simulink model "dcmotor_sim"  (R2020b)
settings: Solver=FixedStepAuto  StartTime=0.0  StopTime=40  FixedStep=Ts  MaxStep=Ts  RelTol=1e-12  AbsTol=1e-6
values from neighbouring files (symbols this model uses):
  Ad = eye(2) + A*Ts    [dcmotor.m]    (also in makedcmotorparams.m)
  Bd = B*Ts    [dcmotor.m]    (also in makedcmotorparams.m)
  C = [1, 1]    [dcmotor.m]    (also in makedcmotorparams.m; tanks.m = [0 1])
  Cd = C    [dcmotor.m]    (also in makedcmotorparams.m)
  delta = 1e-2    (= 0.01)    [dcmotor.m]    (also in makedcmotorparams.m)
  K = place(Ad, Bd, cpoles)    [dcmotor.m]    (also in makedcmotorparams.m)
  L = place(Ad', Cd', [0.6, 0.5]).'    [dcmotor.m]    (also in makedcmotorparams.m = place(Ad', Cd', [0.6, 0]).'; tanks.m = place(A', C', [-100 -2])')
  N = 1/(0.784815)    (= 1.27418563611)    [dcmotor.m]    (also in makedcmotorparams.m = dcgain(T))
  Ts = 1e-3    (= 0.001)    [dcmotor.m]    (also in makedcmotorparams.m)
  x0 = zeros(2,1)    [dcmotor.m]    (also in makedcmotorparams.m)
undefined symbols (not defined in the file or in its folder): AttackPhase
libraries: simulink x1, LinSysLib x1
settings Model: Creator=angelo  LastModifiedBy=angelo

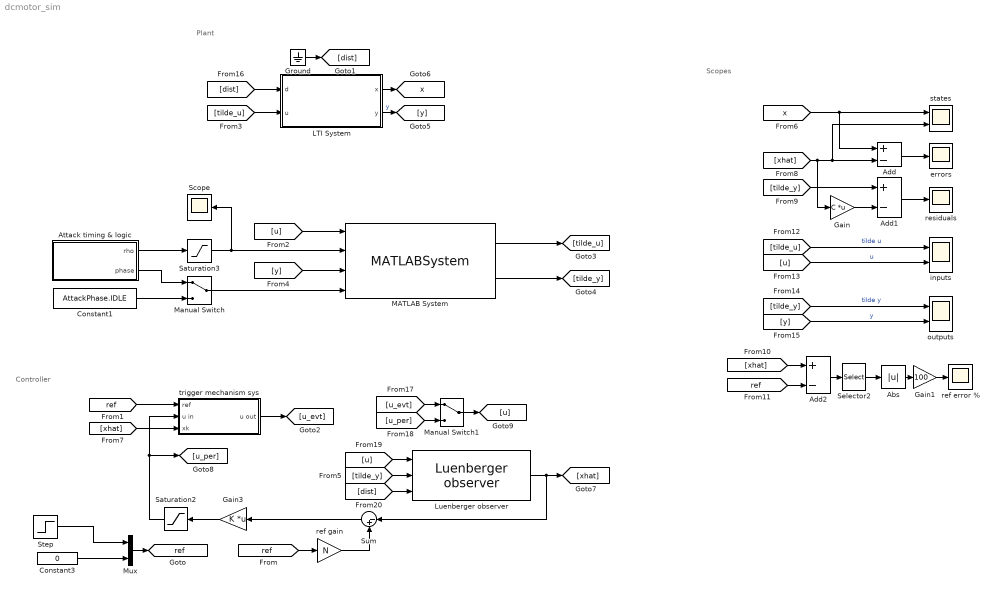
== system dcmotor_sim ==
  note: Scopes
  note: Controller
  note: Plant
  Abs : Abs
  Add : Sum  Inputs=+-
  Add1 : Sum  Inputs=+-
  Add2 : Sum  Inputs=+-
  Attack timing & logic : Subsystem
  Constant1 : Constant  Value=AttackPhase.IDLE
  Constant3 : Constant  Value=0
  Gain : Gain  Gain=C  Multiplication=Matrix(K*u)
  Gain1 : Gain  Gain=100
  Gain3 : Gain  Gain=K  Multiplication=Matrix(K*u)
  Ground : Ground
  LTI System : Subsystem  mask{A=Ad, B=Bd, C=Cd, D=0, x0=x0}
      mask prompts: A "Matrix A:"; B "Matrix B:"; C "Matrix C:"; D "Matrix D:"; x0 "Initial condition:"
      mask help: State space model of an LTI system, with accessible state
      mask Display: disp('DT LTI System')
  Luenberger observer : LinSysLib/Discrete time/Luenberger observer  A=Ad  B=Bd  C=Cd  D=0  hatx0=x0  L=L
  MATLAB System : MATLABSystem  System=ReplayAttacker  bufferSize=1024*1024  SimulateUsing=Code generation
      mask Type: ReplayAttacker
      mask Display:
      | disp('ReplayAttacker');
      | port_label('input',1,'u');
      | port_label('input',2,'rho');
      | port_label('input',3,'y');
      | port_label('input',4,'phase');
      | port_label('output',1,'tildeu');
      | port_label('output',2,'tildey');
  Manual Switch : ManualSwitch
  Manual Switch1 : ManualSwitch
  Mux : Mux  Inputs=2
  Saturation2 : Saturate  UpperLimit=20  LowerLimit=-20
  Saturation3 : Saturate  UpperLimit=20  LowerLimit=-20
  Scope : Scope
  Selector2 : Selector  InputPortWidth=2  IndexOptions=Index vector (dialog)  Indices=1  OutputSizes=1
  Step : Step  Time=0  SampleTime=Ts
  Sum : Sum  Inputs=|-+
  errors : Scope
  inputs : Scope  NumInputPorts=2
  outputs : Scope  NumInputPorts=2
  ref error % : Scope
  ref gain : Gain  Gain=N
  residuals : Scope
  states : Scope  NumInputPorts=2
  trigger mechanism sys : Subsystem
  tag scope: ref=global, x=global
  wires:
  [xhat] -> Gain/1, Add/2, states/2
  [x] -> states/1, Add/1
  Add/1 -> errors/1
  Sum/1 -> Gain3/1
  Mux/1 -> [ref]
  [ref] -> trigger mechanism sys/1(ref)
  LTI System/2(y) -> [y]  "y"
  LTI System/1(x) -> [x]
  [tilde_y] -> Luenberger observer/2
  [xhat] -> trigger mechanism sys/3(xk)
  [tilde_y] -> Add1/1
  Gain/1 -> Add1/2
  Add1/1 -> residuals/1
  Selector2/1 -> Abs/1
  Gain1/1 -> ref error %/1
  Abs/1 -> Gain1/1
  [u] -> MATLAB System/1
  MATLAB System/1 -> [tilde_u]
  MATLAB System/2 -> [tilde_y]
  [y] -> MATLAB System/3
  [u] -> inputs/2  "u"
  [tilde_u] -> inputs/1  "tilde u"
  [tilde_y] -> outputs/1  "tilde y"
  [y] -> outputs/2  "y"
  Manual Switch/1 -> MATLAB System/4
  Constant1/1 -> Manual Switch/2
  trigger mechanism sys/1(u out) -> [u_evt]
  [u_evt] -> Manual Switch1/1
  Gain3/1 -> Saturation2/1
  [u_per] -> Manual Switch1/2
  Manual Switch1/1 -> [u]
  [u] -> Luenberger observer/1
  Constant3/1 -> Mux/2
  [ref] -> ref gain/1
  [xhat] -> Add2/1
  [ref] -> Add2/2
  Add2/1 -> Selector2/1
  Step/1 -> Mux/1
  ref gain/1 -> Sum/2
  [tilde_u] -> LTI System/2(u)
  Saturation2/1 -> trigger mechanism sys/2(u in), [u_per]
  Attack timing & logic/1(rho) -> Saturation3/1
  Attack timing & logic/2(phase) -> Manual Switch/1
  Saturation3/1 -> MATLAB System/2, Scope/1
  Ground/1 -> [dist]
  [dist] -> LTI System/1(d)
  [dist] -> Luenberger observer/3
  Luenberger observer/1 -> Sum/1, [xhat]

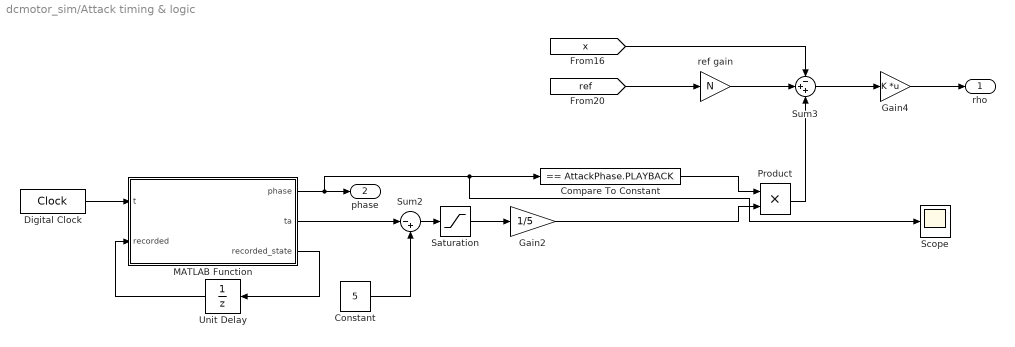
== system dcmotor_sim/Attack timing & logic ==
  Compare To Constant : simulink/Logic and Bit Operations/Compare To Constant  relop===  const=AttackPhase.PLAYBACK  OutDataTypeStr=boolean
  Constant : Constant  Value=5
  Digital Clock : DigitalClock  SampleTime=Ts
  Gain2 : Gain  Gain=1/5
  Gain4 : Gain  Gain=K  Multiplication=Matrix(K*u)
  MATLAB Function : MATLAB Function  TreatAsAtomicUnit=on
  Product : Product
  Saturation : Saturate  UpperLimit=inf  LowerLimit=0
  Scope : Scope
  Sum2 : Sum  Inputs=|-+
  Sum3 : Sum  Inputs=-++
  Unit Delay : UnitDelay  SampleTime=Ts  HasFrameUpgradeWarning=on
  ref gain : Gain  Gain=N
  rho : Outport
  phase : Outport  Port=2
  wires:
  Sum3/1 -> Gain4/1
  Compare To Constant/1 -> Product/1
  Digital Clock/1 -> MATLAB Function/1(t)
  MATLAB Function/1(phase) -> Scope/1, Compare To Constant/1, phase/1
  Gain2/1 -> Product/2
  MATLAB Function/2(ta) -> Sum2/1
  Gain4/1 -> rho/1
  [ref] -> ref gain/1
  ref gain/1 -> Sum3/2
  Unit Delay/1 -> MATLAB Function/2(recorded)
  Constant/1 -> Sum2/2
  MATLAB Function/3(recorded_state) -> Unit Delay/1
  Product/1 -> Sum3/3
  Saturation/1 -> Gain2/1
  [x] -> Sum3/1
  Sum2/1 -> Saturation/1

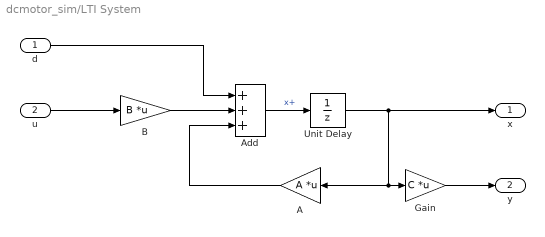
== system dcmotor_sim/LTI System ==
  d : Inport
  u : Inport  Port=2  PortDimensions=size(B,2)
  A : Gain  Gain=A  Multiplication=Matrix(K*u)
  Add : Sum  Inputs=+++
  B : Gain  Gain=B  Multiplication=Matrix(K*u)
  Gain : Gain  Gain=C  Multiplication=Matrix(K*u)
  Unit Delay : UnitDelay  InitialCondition=x0  SampleTime=-1  HasFrameUpgradeWarning=on
  x : Outport  PortDimensions=size(A,1)  VectorParamsAs1DForOutWhenUnconnected=off
  y : Outport  Port=2  PortDimensions=size(C,1)  VectorParamsAs1DForOutWhenUnconnected=off
  wires:
  d/1 -> Add/1
  Gain/1 -> y/1
  A/1 -> Add/3
  Add/1 -> Unit Delay/1  "x+"
  Unit Delay/1 -> Gain/1, A/1, x/1
  B/1 -> Add/2
  u/1 -> B/1

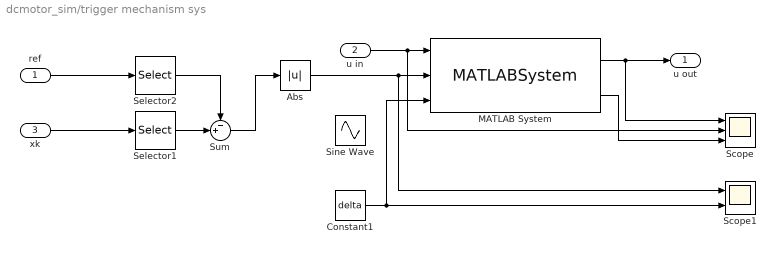
== system dcmotor_sim/trigger mechanism sys ==
  ref : Inport
  u in : Inport  Port=2
  xk : Inport  Port=3
  Abs : Abs
  Constant1 : Constant  Value=delta
  MATLAB System : MATLABSystem  System=TriggerSystem  SimulateUsing=Code generation
      mask Type: TriggerSystem
      mask Display:
      | disp('TriggerSystem');
      | port_label('input',1,'u');
      | port_label('input',2,'err');
      | port_label('input',3,'delta');
      | port_label('output',1,'uTrig');
      | port_label('output',2,'trig');
  Scope : Scope  NumInputPorts=3
  Scope1 : Scope  NumInputPorts=2
  Selector1 : Selector  InputPortWidth=2  IndexOptions=Index vector (dialog)  Indices=1  OutputSizes=1
  Selector2 : Selector  InputPortWidth=2  IndexOptions=Index vector (dialog)  Indices=1  OutputSizes=1
  Sine Wave : Sin  Amplitude=delta  Bias=delta  SampleTime=Ts
  Sum : Sum  Inputs=-+|
  u out : Outport
  wires:
  u in/1 -> Scope/2, MATLAB System/1
  Abs/1 -> Scope1/1, MATLAB System/2
  xk/1 -> Selector1/1
  Sum/1 -> Abs/1
  Selector1/1 -> Sum/2
  Selector2/1 -> Sum/1
  Constant1/1 -> MATLAB System/3, Scope1/2
  MATLAB System/1 -> Scope/1, u out/1
  MATLAB System/2 -> Scope/3
  ref/1 -> Selector2/1

== matlab function dcmotor_sim/Attack timing & logic/MATLAB Function ==
  data: t input; phase output Enum: AttackPhase size=1; ta output; recorded input; recorded_state output
function [phase, ta, recorded_state] = attackSchedule(t, recorded)

kr = 5;
Tr = 10;
Ta = 10;
ka = 20;

h = mod(t,40);

if h >= kr && h <= kr + Tr && recorded == 0
    phase = AttackPhase.RECORD;
    ta = 10;
    recorded_state = recorded;
elseif h >= ka && h <= ka + Ta
    phase = AttackPhase.PLAYBACK;
    ta = h - ka;
    recorded_state = 1;
else
    phase = AttackPhase.IDLE;
    ta = 10;
    recorded_state = recorded;
end


end
